simulink model "machineModel2"  (R2021a)
settings: Solver=VariableStepAuto  StartTime=0.0  StopTime=10.0  RelTol=1e-3
settings Model: Creator=ibirl  LastModifiedBy=ibirl

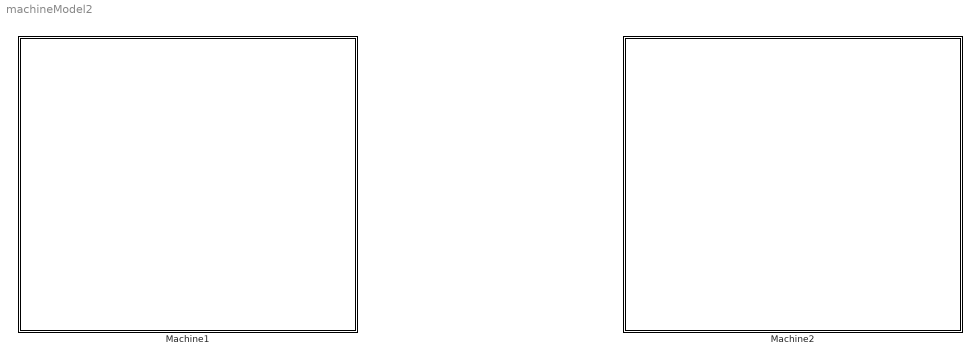
== system machineModel2 ==
  Machine1 : Stateflow chart  TreatAsAtomicUnit=on
  Machine2 : Stateflow chart  TreatAsAtomicUnit=on

== stateflow chart machineModel2/Machine1 ==
  state I
  state H
    (Upstream
    Empty)
  state A
  state B
  state C
  state D
  state E
  state F
  state G
  G -> H [order 3] : [0.020555520000000]{1}
  G -> A [order 2] : [0.657844480000000]{1}
  E -> H [order 3] : [0.013126720000000]{1}
  I -> B [order 2] : [0.779500000000000]{0}
  I -> A [order 1] : [0.210908250000000]{1}
  D -> H [order 3] : [0.009833400000000]{1}
  E -> A [order 4] : [0.393273280000000]{1}
  I -> H [order 3] : [0.009591750000000]{1}
  H -> I [order 2] : [0.021276595744681]{0}
  F -> H [order 4] : [0.013768950000000]{1}
  D -> A [order 4] : [0.354366600000000]{1}
  B -> H [order 3] : [0.016194900000000]{1}
  H -> H [order 1] : [0.978723404255319]{0}
  C -> H [order 4] : [0.013806080000000]{1}
  C -> A [order 3] : [0.525493920000000]{1}
  H -> A [order 3] : [0.021276595744681]{0}
  A -> H [order 3] : [0.009591750000000]{1}
  B -> A [order 2] : [0.421505100000000]{1}
  C -> D [order 1] : [0.276800000000000]{0}
  B -> C [order 4] : [0.346000000000000]{0}
  D -> E [order 1] : [0.343000000000000]{0}
  E -> F [order 1] : [0.352600000000000]{0}
  F -> G [order 1] : [0.380200000000000]{0}
  A -> A [order 2] : [0.210908250000000]{1}
  F -> A [order 3] : [0.385331050000000]{1}
  A -> B [order 1] : [0.779500000000000]{0}
  B -> B [order 1] : [0.2163]{0}
  C -> C [order 2] : Comment *C* [0.1839]{0}
  D -> D [order 2] : [0.2928]{0}
  E -> E [order 2] : [0.241]{0}
  F -> F [order 2] : [0.2207]{0}
  G -> G [order 1] : [0.3216]{0}

== stateflow chart machineModel2/Machine2 ==
  state f
  state e
  state a
  state b
  state c
  state d
  f -> b [order 2] : [0.586200000000000]{0}
  d -> e [order 3] : [0.029074080000000]{-1}
  f -> a [order 1] : [0.392034120000000]{-1}
  f -> e [order 3] : [0.021765880000000]{-1}
  e -> f [order 2] : [0.019607843137255]{0}
  d -> a [order 2] : [0.581725920000000]{-1}
  b -> e [order 3] : [0.045758160000000]{-1}
  e -> e [order 1] : [0.980392156863]{0}
  c -> e [order 3] : [0.040003380000000]{-1}
  c -> a [order 2] : [0.480196620000000]{-1}
  e -> a [order 3] : (1)[0.019607843137255]{0}
  a -> e [order 3] : [0.021765880000000]{-1}
  b -> a [order 2] : [0.732441840000000]{-1}
  b -> c [order 4] : [0.082900000000000]{0}
  c -> d [order 4] : [0.238500000000000]{0}
  a -> a [order 2] : [0.392034120000000]{-1}
  a -> b [order 1] : [0.586200000000000]{0}
  b -> b [order 1] : [0.138900000000000]{0}
  c -> c [order 1] : [0.241300000000000]{0}
  d -> d [order 1] : [0.389200000000000]{0}
